simulink model "model_qam_64_upsampled_2023a"  (R2023a)
settings: Solver=FixedStepDiscrete  StartTime=0.0  StopTime=inf  RelTol=1e-3
libraries: commdigbbndam3 x2, commchan3 x1, commrandsrc3 x1, commsink2 x1, dspsigops x1
settings Model: Creator=D.mon  LastModifiedBy=D.mon
settings RTWCC: GPUComputeCapability=5.0
settings ConfigComp: CovBoundaryAbsTol=1.0e-5

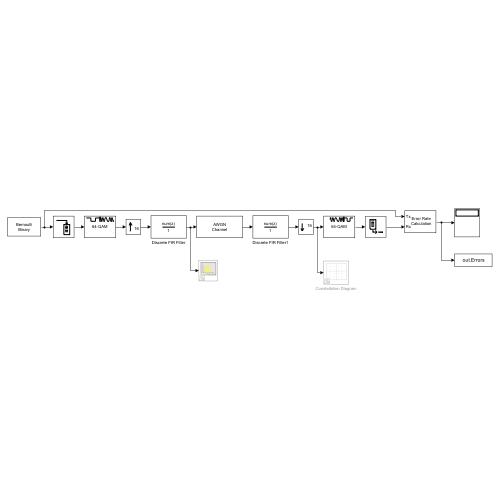
[thumbnail: Simulink's stored preview of the top-level diagram]
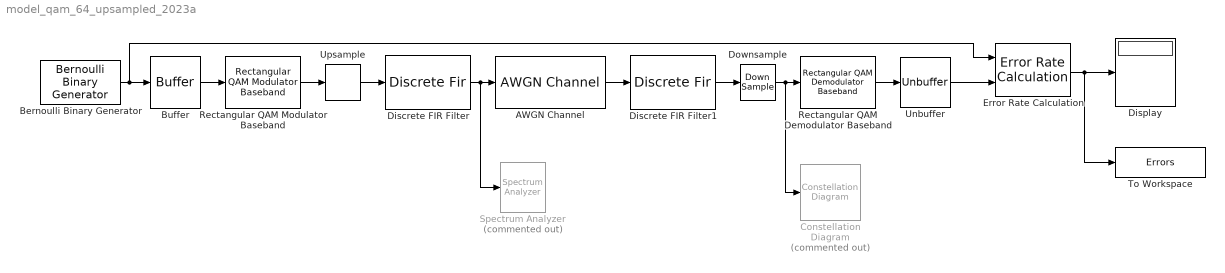
== system model_qam_64_upsampled_2023a ==
  AWGN Channel : commchan3/AWGN Channel  LegacyMode=off  NoiseMethod="Signal to noise ratio  (Eb/No)"  noiseMode="Signal to noise ratio  (SNR)"  EbNo=EbPerNo  EsNo=10  SNR=10  BitsPerSymbol=6  SignalPower=1  SamplesPerSymbol=16  SymbolPeriod=1  VarianceSource=Parameter  Variance=1  RandomStream=mt19937ar with seed  Seed=randi(100000)  SimulateUsing=Code generation
  Bernoulli Binary Generator : commrandsrc3/Bernoulli Binary Generator  ProbabilityOfZero=0.5  SeedSource=Auto  Seed=0  SampleTime=1  SamplesPerFrame=1  OutputDataType=double  SimulateUsing=Interpreted execution
  Buffer : Buffer  N=6  OutputFrames=off
  Constellation Diagram : ConstellationDiagram  Commented=on  WindowPosition=[724.000000,230.000000,600.000000,596.000000,]  Visible=on  ScopeFrameLocation=window  SamplesPerSymbol=4  SymbolsToDisplaySource=Property  SymbolsToDisplay=400  ReferenceConstellation=QPSK  ShowReferenceConstellation=off
  Discrete FIR Filter : DiscreteFir  Coefficients=rcosdesign(1, 6, 16, 'sqrt')*4  InputProcessing=Columns as channels (frame based)
  Discrete FIR Filter1 : DiscreteFir  Coefficients=rcosdesign(1, 6, 16, 'sqrt')/4  InputProcessing=Columns as channels (frame based)
  Display : Display
  Downsample : DownSample  N=16  RateOptions=Allow multirate processing  AllowArbitraryFixedInput=on
  Error Rate Calculation : commsink2/Error Rate Calculation  N=42  st_delay=0  cp_mode=Entire frame  subframe=[]  PMode=Port  WsName=Errors  RsMode2=off  stop=on  numErr=1000  maxBits=1e6
  Rectangular QAM Demodulator Baseband : commdigbbndam3/Rectangular QAM Demodulator Baseband  M=64  OutType=Bit  DecType=Hard decision  VarSource=Dialog  Variance=1  Dec=Gray  Mapping=[0:15]  PowType=Average Power  MinDist=2  AvgPow=1  PeakPow=1  Ph=0  outDtype1=Inherit via internal rule  outDtype2=Inherit via internal rule  derotateFactorWordLen=16  derotateFactorDataTypeStr=Inherit: Same word length as input  derotateFactorLastDataTypeStr=Inherit: Same word length as input  denormFactorWordLen=16  denormFactorDataTypeStr=Inherit: Same word length as input  denormFactorLastDataTypeStr=Inherit: Same word length as input  prodOutWordLen=32  prodOutOverflowMode=Wrap  prodOutRoundingMode=Floor  prodOutOvFlMode=off  prodOutOvFlModeLastStrValue=off  sumWordLen=32
  Rectangular QAM Modulator Baseband : commdigbbndam3/Rectangular QAM Modulator Baseband  M=64  InType=Bit  Enc=Gray  Mapping=[0:15]  PowType=Average Power  MinDist=2  AvgPow=1  PeakPow=1  Ph=0  outDtype=double  outWordLen=16  outUDDataType=sfix(16)  outFracLenMode=Best precision  outFracLen=15  outDataTypeStr=double  outLastDataTypeStr=double
  Spectrum Analyzer : SpectrumAnalyzer  Commented=on  WindowPosition=[808.000000,377.000000,800.000000,500.000000,]  ScopeFrameLocation=window  Span=2.6666666666666665  StartFrequency=-1.3333333333333333  StopFrequency=1.3333333333333333  YLimits=[-59.4194 20.7182]  ExpandToolstrip=on
  To Workspace : ToWorkspace  VariableName=Errors  SampleTime=-1
      settings: MaxDataPoints=1
  Unbuffer : Unbuffer
  Upsample : dspsigops/Upsample  FactorSource=Dialog parameter  N=16  Nmax=16  phase=0  InputProcessing=Columns as channels (frame based)  RateOptions=Allow multirate processing  ic=0  mode=Unused parameter value
  wires:
  Bernoulli Binary Generator/1 -> Error Rate Calculation/1, Buffer/1
  Buffer/1 -> Rectangular QAM Modulator Baseband/1
  Rectangular QAM Modulator Baseband/1 -> Upsample/1
  Rectangular QAM Demodulator Baseband/1 -> Unbuffer/1
  Unbuffer/1 -> Error Rate Calculation/2
  Error Rate Calculation/1 -> Display/1, To Workspace/1
  Downsample/1 -> Constellation Diagram/1, Rectangular QAM Demodulator Baseband/1
  Discrete FIR Filter/1 -> Spectrum Analyzer/1, AWGN Channel/1
  Upsample/1 -> Discrete FIR Filter/1
  AWGN Channel/1 -> Discrete FIR Filter1/1
  Discrete FIR Filter1/1 -> Downsample/1
